simulink model "control_robust_second_order_inversion_algorithms_2018"  (Simulink 10.0)
settings: Solver=VariableStepAuto  StartTime=0.0  StopTime=4  RelTol=1e-3
undefined symbols (not defined in the file or in its folder): DiscIntNeverNeededParam, q0, q0_dot, Tc
settings Model: LogicAnalyzerSignalOrdering=b4b32ae8-4ec4-4001-8231-8f2a4b108c1f,74f067ee-4678-4d5a-844c-a2c6a774325a,bc7b625d-9165-40f1-a33d-a557542bf9b1,12ef16df-f611-4289-9c30-3cd9086cbfa3  Creator=swl782203812  LastModifiedBy=Administrator
settings DataIOCC: SaveFormat=Dataset  ReturnWorkspaceOutputs=on
settings OptimizationCC: LifeSpan=auto
settings DebuggingCC: UnderspecifiedInitializationDetection=Simplified  MergeDetectMultiDrivingBlocksExec=error  SFUnexpectedBacktrackingDiag=error  SFNoUnconditionalDefaultTransitionDiag=error  SFExecutionAtInitializationDiag=warning
settings HardwareCC: ProdBitPerPointer=64  ProdBitPerSizeT=64  ProdBitPerPtrDiffT=64  ProdLargestAtomicFloat=Float  ProdIntDivRoundTo=Zero  ProdEndianess=LittleEndian  ProdWordSize=64  ProdHWDeviceType=Intel->x86-64 (Windows64)
settings ModelReferenceCC: PropagateSignalLabelsOutOfModel=on
settings SFSimCC: SimUseLocalCustomCode=on
settings RTWCC: RTWUseLocalCustomCode=on
settings CodeAppCC: StateflowObjectComments=off
settings GRTTargetCC: TargetLangStandard=C99 (ISO)  CombineOutputUpdateFcns=on  GRTInterface=off
settings ConfigComp: CovMetricSettings=dwe  CovHtmlReporting=off  CovSaveCumulativeToWorkspaceVar=off  CovSaveSingleToWorkspaceVar=off

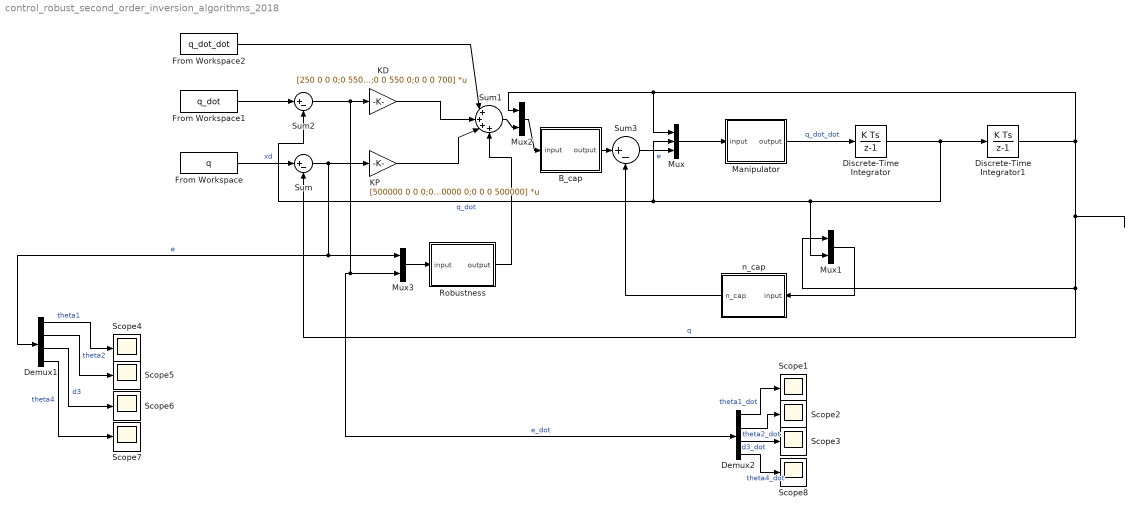
== system control_robust_second_order_inversion_algorithms_2018 ==
  B_cap : MATLAB Function  TreatAsAtomicUnit=on
  Demux1 : Demux
  Demux2 : Demux
  Discrete-Time Integrator : DiscreteIntegrator  InitialCondition=q0_dot  SampleTime=Tc  ICPrevOutput=DiscIntNeverNeededParam  ICPrevScaledInput=DiscIntNeverNeededParam
  Discrete-Time Integrator1 : DiscreteIntegrator  InitialCondition=q0  SampleTime=Tc  ICPrevOutput=DiscIntNeverNeededParam  ICPrevScaledInput=DiscIntNeverNeededParam
  From Workspace : FromWorkspace  VariableName=q  SampleTime=Tc
  From Workspace1 : FromWorkspace  VariableName=q_dot  SampleTime=Tc
  From Workspace2 : FromWorkspace  VariableName=q_dot_dot  SampleTime=Tc
  KD : Gain  Gain=[250 0 0 0;0 550 0 0;0 0 550 0;0 0 0 700]  Multiplication=Matrix(K*u) (u vector)
  KP : Gain  Gain=[500000 0 0 0;0 500000 0 0;0 0 500000 0;0 0 0 500000]  Multiplication=Matrix(K*u) (u vector)
  Manipulator : MATLAB Function  TreatAsAtomicUnit=on
  Mux : Mux  Inputs=3
  Mux1 : Mux  Inputs=2
  Mux2 : Mux  Inputs=2
  Mux3 : Mux  Inputs=2
  Robustness : MATLAB Function  TreatAsAtomicUnit=on
  Scope{1..8} (8 alike) : Scope
  Sum : Sum  Inputs=|+-
  Sum1 : Sum  Inputs=|++++
  Sum2 : Sum  Inputs=|+-
  Sum3 : Sum  Inputs=|+-
  n_cap : MATLAB Function  TreatAsAtomicUnit=on
  wires:
  From Workspace/1 -> Sum/1  "xd"
  Sum/1 -> KP/1, Mux3/1, Demux1/1  "e"
  Discrete-Time Integrator/1 -> Discrete-Time Integrator1/1, Mux1/2, Mux/2, Sum2/2  "q_dot"
  From Workspace1/1 -> Sum2/1
  KP/1 -> Sum1/3
  Manipulator/1(output) -> Discrete-Time Integrator/1  "q_dot_dot"
  Mux/1 -> Manipulator/1(input)
  From Workspace2/1 -> Sum1/1
  Sum2/1 -> KD/1, Demux2/1, Mux3/2  "e_dot"
  Discrete-Time Integrator1/1 -> Sum/2, Mux1/1, Mux2/1, Mux/1  "q"
  Mux1/1 -> n_cap/1(input)
  KD/1 -> Sum1/2
  Demux1/1 -> Scope4/1  "theta1"
  Demux1/2 -> Scope5/1  "theta2"
  Demux1/3 -> Scope6/1  "d3"
  Demux1/4 -> Scope7/1  "theta4"
  Sum3/1 -> Mux/3  "e"
  B_cap/1(output) -> Sum3/1
  Mux2/1 -> B_cap/1(input)
  Sum1/1 -> Mux2/2
  n_cap/1(n_cap) -> Sum3/2
  Mux3/1 -> Robustness/1(input)
  Robustness/1(output) -> Sum1/4
  Demux2/1 -> Scope1/1  "theta1_dot"
  Demux2/2 -> Scope2/1  "theta2_dot"
  Demux2/3 -> Scope3/1  "d3_dot"
  Demux2/4 -> Scope8/1  "theta4_dot"

== matlab function Manipulator ==
  data: input input double; output output double
function output = Manipulator(input)
% Part 2 manipulator
    theta1 = input(1,:);
    theta2 = input(2,:);
    d3 = input(3,:);
    theta4 = input(4,:);
    theta1_dot = input(5,:);
    theta2_dot = input(6,:);
    d3_dot = input(7,:);
    theta4_dot = input(8,:);
    u1 = input(9,:);
    u2 = input(10,:);
    u3 = input(11,:);
    u4 = input(12,:);
    m_l1 = 25;
    m_l2 = 25;
    m_l3 = 10;
    m_l4 = 5;
    I_l1 = 5;
    I_l2 = 5;
    I_l4 = 1;
    I_m1 = 0.0001;
    I_m2 = 0.0001;
    I_m3 = 0.01;
    I_m4 = 0.005;
    l_1 = 0.25;
    l_2 = 0.25;
    k_r1 = 1;
    k_r2 = 1;
    k_r3 = 50;
    k_r4 = 20;
    g = 9.8;
    Fv_1 = 0.0001;
    Fv_2 = 0.0001;
    Fv_3 = 0.01;
    Fv_4 = 0.005;
    
    b11=l_1^2*m_l1+(0.25+l_2^2+l_2*cos(theta2))*m_l2+(0.5+0.5*cos(theta2))*(m_l3+m_l4)+I_l1+I_l2+I_l4+I_m1*k_r1^2+I_m2+I_m3+I_m4;
    b12=(0.5*l_2*cos(theta2)+l_2^2)*m_l2+(0.25+0.25*cos(theta2))*(m_l3+m_l4)+I_l2+I_l4+I_m2*k_r2++I_m3+I_m4;
    b13=-k_r3*I_m3;
    b14=k_r4*I_m4+I_l4;
    b21=b12;
    b22=l_2^2*m_l2+0.25*(m_l4+m_l3)+I_l2+I_l4+I_m2*k_r2^2+I_m4+I_m3;
    b23=-k_r3*I_m3;
    b24=k_r4*I_m4+I_l4;
    b31=b13;
    b32=b23;
    b33=I_m3*k_r3^2+m_l3+m_l4;
    b34=0;
    b41=b14;
    b42=b24;
    b43=b34;
    b44=I_m4*k_r4^2+I_l4;
    B=[b11 b12 b13 b14; b21 b22 b23 b24; b31 b32 b33 b34; b41 b42 b43 b44];
    C=[(-l_2*m_l2*sin(theta2)-0.5*(m_l4+m_l3)*sin(theta2))/2*theta2_dot (-l_2*m_l2*sin(theta2)-0.5*(m_l4+m_l3)*sin(theta2))/2*(theta1_dot+theta2_dot) 0 0;
    -(-l_2*m_l2*sin(theta2)-0.5*(m_l4+m_l3)*sin(theta2))/2*theta1_dot 0 0 0; 0 0 0 0; 0 0 0 0];
    G = [0; 0; -(m_l3+m_l4)*g; 0];
    F = diag([k_r1^2*Fv_1 k_r2^2*Fv_2 k_r3^2*Fv_3 k_r4^2*Fv_4]);
    
    tou = [u1 u2 u3 u4]';
    tou_1 = C*[theta1_dot theta2_dot d3_dot theta4_dot]'+F*[theta1_dot theta2_dot d3_dot theta4_dot]'+G;
    
    q_dot_dot = inv(B)*(tou-tou_1);
    
    output = q_dot_dot;
    % output(2) = q_dot_dot(2);
    % output(3) = q_dot_dot(3);
    % output(4) = q_dot_dot(4);
end

== matlab function B_cap ==
  data: input input double; output output double
function output  = B_cap(input)
    theta2=input(2,:);
    y1=input(5,:);
    y2=input(6,:);
    y3=input(7,:);    
    y4=input(8,:);
    m_l1 = 25;
    m_l2 = 25;
    m_l3 = 10;
    m_l4 = 0;
    I_l1 = 5;
    I_l2 = 5;
    I_l4 = 1;
    I_m1 = 0.0001;
    I_m2 = 0.0001;
    I_m3 = 0.01;
    I_m4 = 0.005;
    l_1 = 0.25;
    l_2 = 0.25;
    k_r1 = 1;
    k_r2 = 1;
    k_r3 = 50;
    k_r4 = 20;
    g = 9.8;
    b11=l_1^2*m_l1+(0.25+l_2^2+l_2*cos(theta2))*m_l2+(0.5+0.5*cos(theta2))*(m_l3+m_l4)+I_l1+I_l2+I_l4+I_m1*k_r1^2+I_m2+I_m3+I_m4;
    b12=(0.5*l_2*cos(theta2)+l_2^2)*m_l2+(0.25+0.25*cos(theta2))*(m_l3+m_l4)+I_l2+I_l4+I_m2*k_r2++I_m3+I_m4;
    b13=-k_r3*I_m3;
    b14=k_r4*I_m4+I_l4;
    b21=b12;
    b22=l_2^2*m_l2+0.25*(m_l4+m_l3)+I_l2+I_l4+I_m2*k_r2^2+I_m4+I_m3;
    b23=-k_r3*I_m3;
    b24=k_r4*I_m4+I_l4;
    b31=b13;
    b32=b23;
    b33=I_m3*k_r3^2+m_l3+m_l4;
    b34=0;
    b41=b14;
    b42=b24;
    b43=b34;
    b44=I_m4*k_r4^2+I_l4;
    B_cap=[b11 b12 b13 b14; b21 b22 b23 b24; b31 b32 b33 b34; b41 b42 b43 b44];
    output=B_cap*[y1 y2 y3 y4]';
end

== matlab function n_cap ==
  data: input input double; n_cap output double
function n_cap  = n_cap(input)
    theta2=input(2,:);
    theta1_dot=input(5,:);
    theta2_dot=input(6,:);
    d3_dot=input(7,:);
    theta4_dot=input(8,:);
    m_l2 = 25;
    m_l3 = 10;
    m_l4 = 0;
    l_2 = 0.25;
    k_r1 = 1;
    k_r2 = 1;
    k_r3 = 50;
    k_r4 = 20;
    g = 9.8;
    Fv_1 = 0.0001;
    Fv_2 = 0.0001;
    Fv_3 = 0.01;
    Fv_4 = 0.005;
    C_cap=[(-l_2*m_l2*sin(theta2)-0.5*(m_l4+m_l3)*sin(theta2))/2*theta2_dot (-l_2*m_l2*sin(theta2)-0.5*(m_l4+m_l3)*sin(theta2))/2*(theta1_dot+theta2_dot) 0 0;
    -(-l_2*m_l2*sin(theta2)-0.5*(m_l4+m_l3)*sin(theta2))/2*theta1_dot 0 0 0; 0 0 0 0; 0 0 0 0];
    G = [0; 0; -(m_l3+m_l4)*g; 0];
    F = diag([k_r1^2*Fv_1 k_r2^2*Fv_2 k_r3^2*Fv_3 k_r4^2*Fv_4]);
    n_cap = C_cap*[theta1_dot theta2_dot d3_dot theta4_dot]'+F*[theta1_dot theta2_dot d3_dot theta4_dot]'+G;
end

== matlab function Robustness ==
  data: input input double; output output double
function output  = Robustness(input)
%ROBUSTENESS Summary of this function goes here
%   Detailed explanation goes here
e_1=input(1);
e_2=input(2);
e_3=input(3);
e_4=input(4);
e_1_dot=input(5);
e_2_dot=input(6);
e_3_dot=input(7);
e_4_dot=input(8);
D=[zeros(4,4) eye(4)]';
Q=eye(8);
zita=[e_1 e_2 e_3 e_4 e_1_dot e_2_dot e_3_dot e_4_dot]';
z=D'*Q*zita;
n_z=norm(z,2);
epsilon=0.06;
ro=70;
if n_z>=epsilon
    output=ro*z/n_z;
else
    output=ro*z/epsilon;
end
